simulink library "LIB_CycleControl"  (R2018b)
settings: Solver=VariableStepAuto  StartTime=0.0  StopTime=10.0  RelTol=1e-3
undefined symbols (not defined in the file or in its folder): eActuators, eRespiratorStates, NActuatorActive, nBlowerCmdInit, nBlowerCmdMax, nBlowerCmdMin, nBlowerDecHigh, nBlowerDecMedium, nBlowerIncHigh, nBlowerIncLow, nBlowerIncMedium, NBlowerSpeedIncCorrectionGain, NBlowerValveDerivativeGain, NBlowerValveIntegralGain, NBlowerValveIntegralHighGain, NBlowerValvePropGain, NCyclePerMinMax, NCyclePerMinMin, NMaxPressureSample, NPatientValveDerivativeGain, NPatientValveIntegralGain, NPatientValveIntegralHighGain, NPatientValvePropGain, pBlowerValveOutletOffset, pDiffMaxThdForPlateauPlausibility, pDiffThdForBlowerValveControlActivation, pDiffThdForPatientValveControlActivation, pErrorPlausibilityThd, pErrorThdForHighBlowerDec, pStaticErrorThdForHighBlowerInc, rPIDIntegralMaxTermForBlowerValve, rPIDIntegralMaxTermForPatientValve, rPIDIntegralMinTermForBlowerValve, rPIDIntegralMinTermForPatientValve, tBlowerValveOpen, tDelayBeforeRespiratorCycleStart, tDelayForRespiratorStop, tPatientValveOpen, tPhase1Ofs, tStopInhalationPhase1Min
libraries: simulink x62, simulink_need_slupdate x4, simulink_extras x3
(part 1 of 4)
settings Model: Creator=BRAUL  LastModifiedBy=VITIE

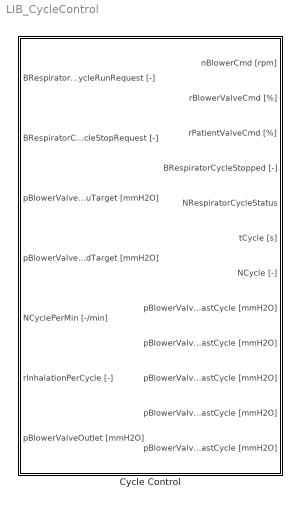
== system LIB_CycleControl ==
  Cycle Control : Subsystem
      settings: AttributesFormatString=%<ReferenceBlock>

== system LIB_CycleControl/Cycle Control ==
  BRespiratorCycleRunRequest [-] : Inport
  BRespiratorCycleStopRequest [-] : Inport  Port=2
  pBlowerValveOutletPlateauTarget [mmH2O] : Inport  Port=3  OutDataTypeStr=single
  pBlowerValveOutletEndTarget [mmH2O] : Inport  Port=4  OutDataTypeStr=single
  NCyclePerMin [-/min] : Inport  Port=5  OutDataTypeStr=single
  rInhalationPerCycle [-] : Inport  Port=6  OutDataTypeStr=single
  pBlowerValveOutlet [mmH2O] : Inport  Port=7  OutDataTypeStr=single
  Compare To Constant : simulink/Logic and Bit Operations/Compare To Constant  relop===  const=eActuators.None  OutDataTypeStr=boolean
  Constant9 : Constant  Value=NActuatorActive  VectorParams1D=off  OutDataTypeStr=Enum: eActuators
  Cycle Control Wrapper : Subsystem
  nBlowerCmd [rpm] : Outport  OutDataTypeStr=single
  rBlowerValveCmd [%] : Outport  Port=2  OutDataTypeStr=single
  rPatientValveCmd [%] : Outport  Port=3  OutDataTypeStr=single
  BRespiratorCycleStopped [-] : Outport  Port=4  OutDataTypeStr=boolean  InitialOutput=0
  NRespiratorCycleStatus : Outport  Port=5
  tCycle [s] : Outport  Port=6
  NCycle [-] : Outport  Port=7
  pBlowerValveOutletPeakLastCycle [mmH2O] : Outport  Port=8
  pBlowerValveOutletPlateauLastCycle [mmH2O] : Outport  Port=9  InitialOutput=0
  pBlowerValveOutletEndLastCycle [mmH2O] : Outport  Port=10
  pBlowerValveOutletPlateauTargetAppliedLastCycle [mmH2O] : Outport  Port=11
  pBlowerValveOutletEndTargetAppliedLastCycle [mmH2O] : Outport  Port=12
  wires:
  Cycle Control Wrapper/7(NCycle [-]) -> NCycle [-]/1
  Cycle Control Wrapper/9(pBlowerValveOutletPlateauLastCycle [mmH2O]) -> pBlowerValveOutletPlateauLastCycle [mmH2O]/1
  Cycle Control Wrapper/8(pBlowerValveOutletPeakLastCycle [mmH2O]) -> pBlowerValveOutletPeakLastCycle [mmH2O]/1
  Cycle Control Wrapper/11(pBlowerValveOutletPlateauTargetAppliedLastCycle [mmH2O]) -> pBlowerValveOutletPlateauTargetAppliedLastCycle [mmH2O]/1
  Cycle Control Wrapper/12(pBlowerValveOutletEndTargetAppliedLastCycle [mmH2O]) -> pBlowerValveOutletEndTargetAppliedLastCycle [mmH2O]/1
  Cycle Control Wrapper/10(pBlowerValveOutletEndLastCycle [mmH2O]) -> pBlowerValveOutletEndLastCycle [mmH2O]/1
  Cycle Control Wrapper/5(NRespiratorCycleStatus) -> NRespiratorCycleStatus/1
  Cycle Control Wrapper/6(tCycle [s]) -> tCycle [s]/1
  BRespiratorCycleStopRequest [-]/1 -> Cycle Control Wrapper/2(BRespiratorCycleStopRequest [-])
  BRespiratorCycleRunRequest [-]/1 -> Cycle Control Wrapper/1(BRespiratorCycleRunRequest [-])
  Cycle Control Wrapper/4(BRespiratorCycleStopped [-]) -> BRespiratorCycleStopped [-]/1
  Cycle Control Wrapper/1(nBlowerCmd [rpm]) -> nBlowerCmd [rpm]/1
  Cycle Control Wrapper/2(rBlowerValveCmd [%]) -> rBlowerValveCmd [%]/1
  Cycle Control Wrapper/3(rPatientValveCmd [%]) -> rPatientValveCmd [%]/1
  pBlowerValveOutletPlateauTarget [mmH2O]/1 -> Cycle Control Wrapper/3(pBlowerValveOutletPlateauTarget [mmH2O])
  pBlowerValveOutletEndTarget [mmH2O]/1 -> Cycle Control Wrapper/4(pBlowerValveOutletEndTarget [mmH2O])
  NCyclePerMin [-/min]/1 -> Cycle Control Wrapper/5(NCyclePerMin [-/min])
  rInhalationPerCycle [-]/1 -> Cycle Control Wrapper/6(rInhalationPerCycle [-])
  pBlowerValveOutlet [mmH2O]/1 -> Cycle Control Wrapper/7(pBlowerValveOutlet [mmH2O])
  Compare To Constant/1 -> Cycle Control Wrapper/Enable
  Constant9/1 -> Compare To Constant/1

== system LIB_CycleControl/Cycle Control/Cycle Control Wrapper ==
  BRespiratorCycleRunRequest [-] : Inport
  BRespiratorCycleStopRequest [-] : Inport  Port=2
  pBlowerValveOutletPlateauTarget [mmH2O] : Inport  Port=3  OutDataTypeStr=single
  pBlowerValveOutletEndTarget [mmH2O] : Inport  Port=4  OutDataTypeStr=single
  NCyclePerMin [-/min] : Inport  Port=5  OutDataTypeStr=single
  rInhalationPerCycle [-] : Inport  Port=6  OutDataTypeStr=single
  pBlowerValveOutlet [mmH2O] : Inport  Port=7  OutDataTypeStr=single
  Enable : EnablePort  StatesWhenEnabling=reset
  Cycle pController : Subsystem
  nBlowerCmd [rpm] : Outport  OutDataTypeStr=single  InitialOutput=0
  rBlowerValveCmd [%] : Outport  Port=2  OutDataTypeStr=single  InitialOutput=0
  rPatientValveCmd [%] : Outport  Port=3  OutDataTypeStr=single  InitialOutput=0
  BRespiratorCycleStopped [-] : Outport  Port=4  InitialOutput=0
  NRespiratorCycleStatus : Outport  Port=5
  tCycle [s] : Outport  Port=6
  NCycle [-] : Outport  Port=7
  pBlowerValveOutletPeakLastCycle [mmH2O] : Outport  Port=8
  pBlowerValveOutletPlateauLastCycle [mmH2O] : Outport  Port=9  InitialOutput=0
  pBlowerValveOutletEndLastCycle [mmH2O] : Outport  Port=10
  pBlowerValveOutletPlateauTargetAppliedLastCycle [mmH2O] : Outport  Port=11
  pBlowerValveOutletEndTargetAppliedLastCycle [mmH2O] : Outport  Port=12
  wires:
  Cycle pController/7(NCycle [-]) -> NCycle [-]/1
  Cycle pController/11(pBlowerValveOutletEndTargetAppliedLastCycle [mmH2O]) -> pBlowerValveOutletEndTargetAppliedLastCycle [mmH2O]/1
  Cycle pController/12(pBlowerValveOutletPlateauTargetAppliedLastCycle [mmH2O]) -> pBlowerValveOutletPlateauTargetAppliedLastCycle [mmH2O]/1
  Cycle pController/10(pBlowerValveOutletPlateauLastCycle [mmH2O]) -> pBlowerValveOutletPlateauLastCycle [mmH2O]/1
  Cycle pController/9(pBlowerValveOutletEndLastCycle [mmH2O]) -> pBlowerValveOutletEndLastCycle [mmH2O]/1
  Cycle pController/8(pBlowerValveOutletPeakLastCycle [mmH2O]) -> pBlowerValveOutletPeakLastCycle [mmH2O]/1
  Cycle pController/6(tCycle [s]) -> tCycle [s]/1
  Cycle pController/5(NRespiratorCycleStatus) -> NRespiratorCycleStatus/1
  BRespiratorCycleRunRequest [-]/1 -> Cycle pController/1(BRespiratorCycleRunRequest [-])
  BRespiratorCycleStopRequest [-]/1 -> Cycle pController/2(BRespiratorCycleStopRequest [-])
  Cycle pController/4(BRespiratorCycleStopped [-]) -> BRespiratorCycleStopped [-]/1
  pBlowerValveOutletEndTarget [mmH2O]/1 -> Cycle pController/4(pBlowerValveOutletEndTarget [mmH2O])
  Cycle pController/2(rBlowerValveCmd [%]) -> rBlowerValveCmd [%]/1
  Cycle pController/1(nBlowerCmd [rpm]) -> nBlowerCmd [rpm]/1
  NCyclePerMin [-/min]/1 -> Cycle pController/5(NCyclePerMin [-/min])
  pBlowerValveOutletPlateauTarget [mmH2O]/1 -> Cycle pController/3(pBlowerValveOutletPlateauTarget [mmH2O])
  rInhalationPerCycle [-]/1 -> Cycle pController/6(rInhalationPerCycle [-])
  Cycle pController/3(rPatientValveCmd [%]) -> rPatientValveCmd [%]/1
  pBlowerValveOutlet [mmH2O]/1 -> Cycle pController/7(pBlowerValveOutlet [mmH2O])

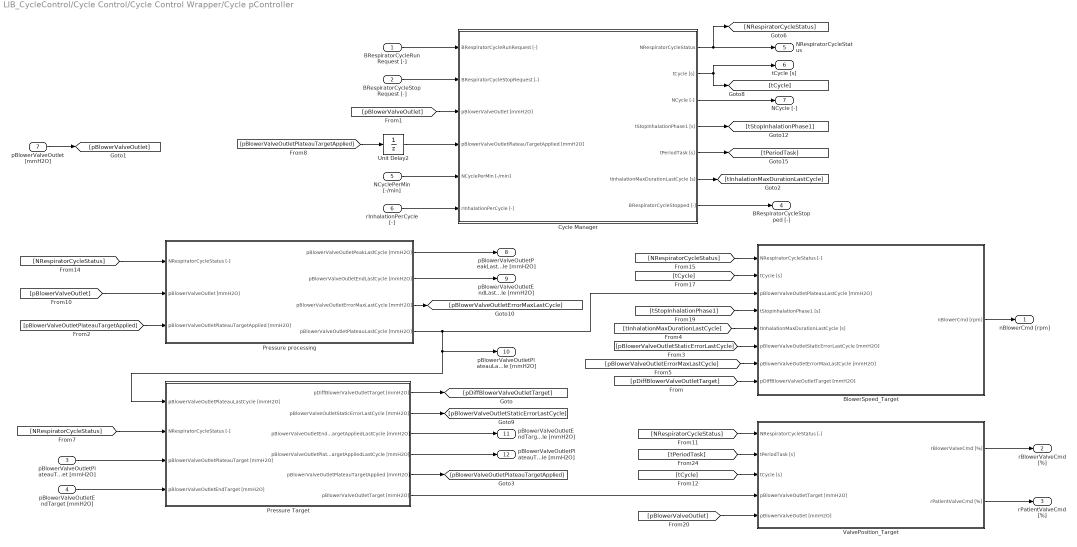
== system LIB_CycleControl/Cycle Control/Cycle Control Wrapper/Cycle pController ==
  BRespiratorCycleRunRequest [-] : Inport
  BRespiratorCycleStopRequest [-] : Inport  Port=2
  pBlowerValveOutletPlateauTarget [mmH2O] : Inport  Port=3
  pBlowerValveOutletEndTarget [mmH2O] : Inport  Port=4
  NCyclePerMin [-/min] : Inport  Port=5
  rInhalationPerCycle [-] : Inport  Port=6
  pBlowerValveOutlet [mmH2O] : Inport  Port=7
  BlowerSpeed_Target : Subsystem
  Cycle Manager : Subsystem
  Pressure Target : Subsystem
  Pressure processing : Subsystem
  Unit Delay2 : UnitDelay  SampleTime=-1
      settings: AttributesFormatString=%<InitialCondition>
  ValvePosition_Target : Subsystem
  nBlowerCmd [rpm] : Outport  InitialOutput=0
  rBlowerValveCmd [%] : Outport  Port=2  InitialOutput=0
  rPatientValveCmd [%] : Outport  Port=3  InitialOutput=0
  BRespiratorCycleStopped [-] : Outport  Port=4  InitialOutput=0
  NRespiratorCycleStatus : Outport  Port=5
  tCycle [s] : Outport  Port=6
  NCycle [-] : Outport  Port=7
  pBlowerValveOutletPeakLastCycle [mmH2O] : Outport  Port=8
  pBlowerValveOutletEndLastCycle [mmH2O] : Outport  Port=9
  pBlowerValveOutletPlateauLastCycle [mmH2O] : Outport  Port=10  InitialOutput=0
  pBlowerValveOutletEndTargetAppliedLastCycle [mmH2O] : Outport  Port=11
  pBlowerValveOutletPlateauTargetAppliedLastCycle [mmH2O] : Outport  Port=12
  wires:
  Cycle Manager/3(NCycle [-]) -> NCycle [-]/1
  Pressure processing/2(pBlowerValveOutletEndLastCycle [mmH2O]) -> pBlowerValveOutletEndLastCycle [mmH2O]/1
  Pressure processing/1(pBlowerValveOutletPeakLastCycle [mmH2O]) -> pBlowerValveOutletPeakLastCycle [mmH2O]/1
  Pressure processing/4(pBlowerValveOutletPlateauLastCycle [mmH2O]) -> BlowerSpeed_Target/3(pBlowerValveOutletPlateauLastCycle [mmH2O]), pBlowerValveOutletPlateauLastCycle [mmH2O]/1, Pressure Target/1(pBlowerValveOutletPlateauLastCycle [mmH2O])
  Pressure processing/3(pBlowerValveOutletErrorMaxLastCycle [mmH2O]) -> [pBlowerValveOutletErrorMaxLastCycle]
  Pressure Target/4(pBlowerValveOutletPlateauTargetAppliedLastCycle [mmH2O]) -> pBlowerValveOutletPlateauTargetAppliedLastCycle [mmH2O]/1
  Pressure Target/3(pBlowerValveOutletEndTargetAppliedLastCycle [mmH2O]) -> pBlowerValveOutletEndTargetAppliedLastCycle [mmH2O]/1
  Pressure Target/5(pBlowerValveOutletPlateauTargetApplied [mmH2O]) -> [pBlowerValveOutletPlateauTargetApplied]
  Pressure Target/1(pDiffBlowerValveOutletTarget [mmH2O]) -> [pDiffBlowerValveOutletTarget]
  [pBlowerValveOutletErrorMaxLastCycle] -> BlowerSpeed_Target/7(pBlowerValveOutletErrorMaxLastCycle [mmH2O])
  [pDiffBlowerValveOutletTarget] -> BlowerSpeed_Target/8(pDiffBlowerValveOutletTarget [mmH2O])
  [pBlowerValveOutletPlateauTargetApplied] -> Pressure processing/3(pBlowerValveOutletPlateauTargetApplied [mmH2O])
  [tCycle] -> ValvePosition_Target/3(tCycle [s])
  BRespiratorCycleRunRequest [-]/1 -> Cycle Manager/1(BRespiratorCycleRunRequest [-])
  BRespiratorCycleStopRequest [-]/1 -> Cycle Manager/2(BRespiratorCycleStopRequest [-])
  Cycle Manager/7(BRespiratorCycleStopped [-]) -> BRespiratorCycleStopped [-]/1
  Cycle Manager/6(tInhalationMaxDurationLastCycle [s]) -> [tInhalationMaxDurationLastCycle]
  Cycle Manager/5(tPeriodTask [s]) -> [tPeriodTask]
  Pressure Target/6(pBlowerValveOutletTarget [mmH2O]) -> ValvePosition_Target/4(pBlowerValveOutletTarget [mmH2O])
  Unit Delay2/1 -> Cycle Manager/4(pBlowerValveOutletPlateauTargetApplied [mmH2O])
  [pBlowerValveOutlet] -> Cycle Manager/3(pBlowerValveOutlet [mmH2O])
  Cycle Manager/4(tStopInhalationPhase1 [s]) -> [tStopInhalationPhase1]
  Cycle Manager/2(tCycle [s]) -> tCycle [s]/1, [tCycle]
  Cycle Manager/1(NRespiratorCycleStatus) -> NRespiratorCycleStatus/1, [NRespiratorCycleStatus]
  rInhalationPerCycle [-]/1 -> Cycle Manager/6(rInhalationPerCycle [-])
  NCyclePerMin [-/min]/1 -> Cycle Manager/5(NCyclePerMin [-/min])
  [pBlowerValveOutletPlateauTargetApplied] -> Unit Delay2/1
  pBlowerValveOutlet [mmH2O]/1 -> [pBlowerValveOutlet]
  [tPeriodTask] -> ValvePosition_Target/2(tPeriodTask [s])
  [pBlowerValveOutletStaticErrorLastCycle] -> BlowerSpeed_Target/6("pBlowerValveOutletStaticErrorLastCycle [mmH2O] ")
  [tInhalationMaxDurationLastCycle] -> BlowerSpeed_Target/5(tInhalationMaxDurationLastCycle [s])
  [tStopInhalationPhase1] -> BlowerSpeed_Target/4(tStopInhalationPhase1 [s])
  Pressure Target/2(pBlowerValveOutletStaticErrorLastCycle [mmH2O]) -> [pBlowerValveOutletStaticErrorLastCycle]
  pBlowerValveOutletPlateauTarget [mmH2O]/1 -> Pressure Target/3(pBlowerValveOutletPlateauTarget [mmH2O])
  [NRespiratorCycleStatus] -> Pressure Target/2(NRespiratorCycleStatus [-])
  pBlowerValveOutletEndTarget [mmH2O]/1 -> Pressure Target/4(pBlowerValveOutletEndTarget [mmH2O])
  [NRespiratorCycleStatus] -> Pressure processing/1(NRespiratorCycleStatus [-])
  [pBlowerValveOutlet] -> Pressure processing/2(pBlowerValveOutlet [mmH2O])
  [pBlowerValveOutlet] -> ValvePosition_Target/5(pBlowerValveOutlet [mmH2O])
  [NRespiratorCycleStatus] -> ValvePosition_Target/1(NRespiratorCycleStatus [-])
  [tCycle] -> BlowerSpeed_Target/2(tCycle [s])
  [NRespiratorCycleStatus] -> BlowerSpeed_Target/1(NRespiratorCycleStatus [-])
  ValvePosition_Target/2(rPatientValveCmd [%]) -> rPatientValveCmd [%]/1
  ValvePosition_Target/1(rBlowerValveCmd [%]) -> rBlowerValveCmd [%]/1
  BlowerSpeed_Target/1(nBlowerCmd [rpm]) -> nBlowerCmd [rpm]/1

== system LIB_CycleControl/Cycle Control/Cycle Control Wrapper/Cycle pController/BlowerSpeed_Target ==
  NRespiratorCycleStatus [-] : Inport
  tCycle [s] : Inport  Port=2
  pBlowerValveOutletPlateauLastCycle [mmH2O] : Inport  Port=3
  tStopInhalationPhase1 [s] : Inport  Port=4
  tInhalationMaxDurationLastCycle [s] : Inport  Port=5
  "pBlowerValveOutletStaticErrorLastCycle [mmH2O] " : Inport  Port=6
  pBlowerValveOutletErrorMaxLastCycle [mmH2O] : Inport  Port=7
  pDiffBlowerValveOutletTarget [mmH2O] : Inport  Port=8
  Compare To Constant1 : simulink/Logic and Bit Operations/Compare To Constant  relop===  const=eRespiratorStates.NRespiratorStart  OutDataTypeStr=boolean
  Compare To Constant2 : simulink/Logic and Bit Operations/Compare To Constant  relop===  const=eRespiratorStates.NRespiratorInInhalationPhase1  OutDataTypeStr=boolean
  Compare To Constant3 : simulink/Logic and Bit Operations/Compare To Constant  relop===  const=eRespiratorStates.NRespiratorStop  OutDataTypeStr=boolean
  CycleStartComputation : Subsystem
  Data Type Conversion : DataTypeConversion
  Detect Increase : simulink/Logic and Bit Operations/Detect Increase  vinit=0.0  OutDataTypeStr=boolean
  If : If  NumInputs=3  IfExpression=u1 ~= 0  ElseIfExpressions=u2 ~= 0,u3 ~= 0  ShowElse=off
  Merge : Merge  Inputs=3  InitialOutput=0
  START : Subsystem
  STOP : Subsystem
  Unit Delay1 : UnitDelay  SampleTime=-1
      settings: AttributesFormatString=%<InitialCondition>
  Unit Delay2 : UnitDelay  SampleTime=-1
      settings: AttributesFormatString=%<InitialCondition>
  nBlowerCmd [rpm] : Outport
  wires:
  Data Type Conversion/1 -> nBlowerCmd [rpm]/1
  pDiffBlowerValveOutletTarget [mmH2O]/1 -> CycleStartComputation/6(pDiffBlowerValveOutletTarget [mmH2O])
  pBlowerValveOutletErrorMaxLastCycle [mmH2O]/1 -> CycleStartComputation/5(pBlowerValveOutletErrorMaxLastCycle [mmH2O])
  CycleStartComputation/1(nBlowerCmd [rpm]) -> Merge/3
  STOP/1(nBlowerCmd [rpm]) -> Merge/2
  [tCycle] -> START/1(tCycle [s])
  If/3 -> CycleStartComputation/Action
  If/2 -> STOP/Action
  Compare To Constant3/1 -> If/2
  Unit Delay2/1 -> CycleStartComputation/2(tStopInhalationPhase1LastCycle [s])
  Merge/1 -> Unit Delay1/1, Data Type Conversion/1
  START/1(nBlowerCmd [rpm]) -> Merge/1
  Detect Increase/1 -> If/3
  If/1 -> START/Action
  Compare To Constant1/1 -> If/1
  Unit Delay1/1 -> CycleStartComputation/7(nBlowerCmdPrev [rpm])
  "pBlowerValveOutletStaticErrorLastCycle [mmH2O] "/1 -> CycleStartComputation/4("pBlowerValveOutletStaticErrorLastCycle [mmH2O] ")
  tInhalationMaxDurationLastCycle [s]/1 -> CycleStartComputation/3(tInhalationMaxDurationLastCycle [s])
  tStopInhalationPhase1 [s]/1 -> Unit Delay2/1
  pBlowerValveOutletPlateauLastCycle [mmH2O]/1 -> CycleStartComputation/1(pBlowerValveOutletPlateauLastCycle [mmH2O])
  NRespiratorCycleStatus [-]/1 -> [NRespiratorCycleStatus]
  [NRespiratorCycleStatus] -> Compare To Constant3/1, Compare To Constant2/1, Compare To Constant1/1
  Compare To Constant2/1 -> Detect Increase/1
  tCycle [s]/1 -> [tCycle]

== system LIB_CycleControl/Cycle Control/Cycle Control Wrapper/Cycle pController/Cycle Manager ==
  BRespiratorCycleRunRequest [-] : Inport
  BRespiratorCycleStopRequest [-] : Inport  Port=2
  pBlowerValveOutlet [mmH2O] : Inport  Port=3
  pBlowerValveOutletPlateauTargetApplied [mmH2O] : Inport  Port=4
  NCyclePerMin [-/min] : Inport  Port=5
  rInhalationPerCycle [-] : Inport  Port=6
  1 : Constant  OutDataTypeStr=single
  Constant3 : Constant  Value=tDelayForRespiratorStop  OutDataTypeStr=single
  Constant4 : Constant  Value=tDelayBeforeRespiratorCycleStart  OutDataTypeStr=single
  Constant9 : Constant  Value=pBlowerValveOutletOffset  OutDataTypeStr=single
  Data Store Write1 : DataStoreWrite  DataStoreName=tCycle
  Data Store Write2 : DataStoreWrite  DataStoreName=NCycle
  Data Store Write3 : DataStoreWrite  DataStoreName=NRespiratorCycleStatus
  Data Store Write4 : DataStoreWrite  DataStoreName=tStopInhalationPhase1
  Data Store Write5 : DataStoreWrite  DataStoreName=BRespiratorCycleStopped
  Respiratory Cycle Management : Stateflow chart  TreatAsAtomicUnit=on
  Timing Setup : Subsystem
  Weighted Sample Time : SampleTimeMath  TsampMathOp=Ts Only  OutDataTypeStr=Inherit: Inherit via back propagation
  NRespiratorCycleStatus : Outport
  tCycle [s] : Outport  Port=2
  NCycle [-] : Outport  Port=3
  tStopInhalationPhase1 [s] : Outport  Port=4
  tPeriodTask [s] : Outport  Port=5
  tInhalationMaxDurationLastCycle [s] : Outport  Port=6
  BRespiratorCycleStopped [-] : Outport  Port=7
  wires:
  Constant3/1 -> Respiratory Cycle Management/10(tDelayForRespiratorStop)
  Constant4/1 -> Respiratory Cycle Management/9(tDelayBeforeRespiratorCycleStart)
  Constant9/1 -> Respiratory Cycle Management/8(pBlowerValveOutletOffset)
  BRespiratorCycleStopRequest [-]/1 -> Respiratory Cycle Management/2(BRespiratorCycleStopRequest)
  BRespiratorCycleRunRequest [-]/1 -> Respiratory Cycle Management/1(BRespiratorCycleRunRequest)
  Respiratory Cycle Management/5(BRespiratorCycleStopped) -> BRespiratorCycleStopped [-]/1, Data Store Write5/1  "BRespiratorCycleStopped"
  Timing Setup/3(tInhalationMaxDurationLastCycle [s]) -> tInhalationMaxDurationLastCycle [s]/1
  Respiratory Cycle Management/1(NRespiratorCycleStatus) -> NRespiratorCycleStatus/1, Data Store Write3/1  "NRespiratorCycleStatus"
  Respiratory Cycle Management/3(NCycle) -> Data Store Write2/1, NCycle [-]/1  "NCycle"
  Timing Setup/2(tInhalationMaxDuration [s]) -> [tInhalationMaxDuration]
  [tInhalationMaxDuration] -> Respiratory Cycle Management/3(tInhalationMaxDuration)
  Respiratory Cycle Management/4(tStopInhalationPhase1) -> tStopInhalationPhase1 [s]/1, Data Store Write4/1  "tStopInhalationPhase1"
  NCyclePerMin [-/min]/1 -> Timing Setup/1(NCyclePerMin [-/min])
  Respiratory Cycle Management/6(fCallCycleComputation()) -> Timing Setup/Trigger
  [tCycleMaxDuration] -> Respiratory Cycle Management/4(tCycleMaxDuration)
  1/1 -> Weighted Sample Time/1
  pBlowerValveOutlet [mmH2O]/1 -> [pBlowerValveOutlet]
  [pBlowerValveOutlet] -> Respiratory Cycle Management/6(pBlowerValveOutlet)
  Timing Setup/1(tCycleMaxDuration [s]) -> [tCycleMaxDuration]
  pBlowerValveOutletPlateauTargetApplied [mmH2O]/1 -> Respiratory Cycle Management/7(pBlowerValveOutletPlateauTargetApplied)
  rInhalationPerCycle [-]/1 -> Timing Setup/2(rInhalationPerCycle [-])
  Respiratory Cycle Management/2(tCycle) -> tCycle [s]/1, Data Store Write1/1  "tCycle"
  Weighted Sample Time/1 -> tPeriodTask [s]/1, Respiratory Cycle Management/5(tSample)

== system LIB_CycleControl/Cycle Control/Cycle Control Wrapper/Cycle pController/Pressure Target ==
  pBlowerValveOutletPlateauLastCycle [mmH2O] : Inport
  NRespiratorCycleStatus [-] : Inport  Port=2
  pBlowerValveOutletPlateauTarget [mmH2O] : Inport  Port=3
  pBlowerValveOutletEndTarget [mmH2O] : Inport  Port=4
  CycleStartComputation : Subsystem
  Data Store Write4 : DataStoreWrite  DataStoreName=pBlowerValveOutletTarget
  InCycleComputation : Subsystem
  pDiffBlowerValveOutletTarget [mmH2O] : Outport
  pBlowerValveOutletStaticErrorLastCycle [mmH2O] : Outport  Port=2
  pBlowerValveOutletEndTargetAppliedLastCycle [mmH2O] : Outport  Port=3
  pBlowerValveOutletPlateauTargetAppliedLastCycle [mmH2O] : Outport  Port=4
  pBlowerValveOutletPlateauTargetApplied [mmH2O] : Outport  Port=5
  pBlowerValveOutletTarget [mmH2O] : Outport  Port=6
  wires:
  CycleStartComputation/1(pDiffBlowerValveOutletTarget [mmH2O]) -> pDiffBlowerValveOutletTarget [mmH2O]/1
  CycleStartComputation/2(pBlowerValveOutletStaticErrorLastCycle [mmH2O]) -> pBlowerValveOutletStaticErrorLastCycle [mmH2O]/1
  CycleStartComputation/4(pBlowerValveOutletPlateauTargetAppliedLastCycle [mmH2O]) -> pBlowerValveOutletPlateauTargetAppliedLastCycle [mmH2O]/1
  CycleStartComputation/3(pBlowerValveOutletEndTargetAppliedLastCycle [mmH2O]) -> pBlowerValveOutletEndTargetAppliedLastCycle [mmH2O]/1
  CycleStartComputation/5(pBlowerValveOutletEndTargetApplied [mmH2O]) -> InCycleComputation/2(pBlowerValveOutletEndTargetApplied [mmH2O])
  [NRespiratorCycleStatus] -> CycleStartComputation/1(NRespiratorCycleStatus [-])
  pBlowerValveOutletEndTarget [mmH2O]/1 -> CycleStartComputation/4(pBlowerValveOutletEndTarget [mmH2O])
  pBlowerValveOutletPlateauTarget [mmH2O]/1 -> CycleStartComputation/2(pBlowerValveOutletPlateauTarget [mmH2O])
  pBlowerValveOutletPlateauLastCycle [mmH2O]/1 -> CycleStartComputation/3(pBlowerValveOutletPlateauLastCycle [mmH2O])
  [NRespiratorCycleStatus] -> InCycleComputation/1(NRespiratorCycleStatus [-])
  CycleStartComputation/6(pBlowerValveOutletPlateauTargetApplied [mmH2O]) -> InCycleComputation/3(pBlowerValveOutletPlateauTargetApplied [mmH2O]), pBlowerValveOutletPlateauTargetApplied [mmH2O]/1
  NRespiratorCycleStatus [-]/1 -> [NRespiratorCycleStatus]
  InCycleComputation/1(pBlowerValveOutletTarget [mmH2O]) -> pBlowerValveOutletTarget [mmH2O]/1, Data Store Write4/1  "pBlowerValveOutletTarget"

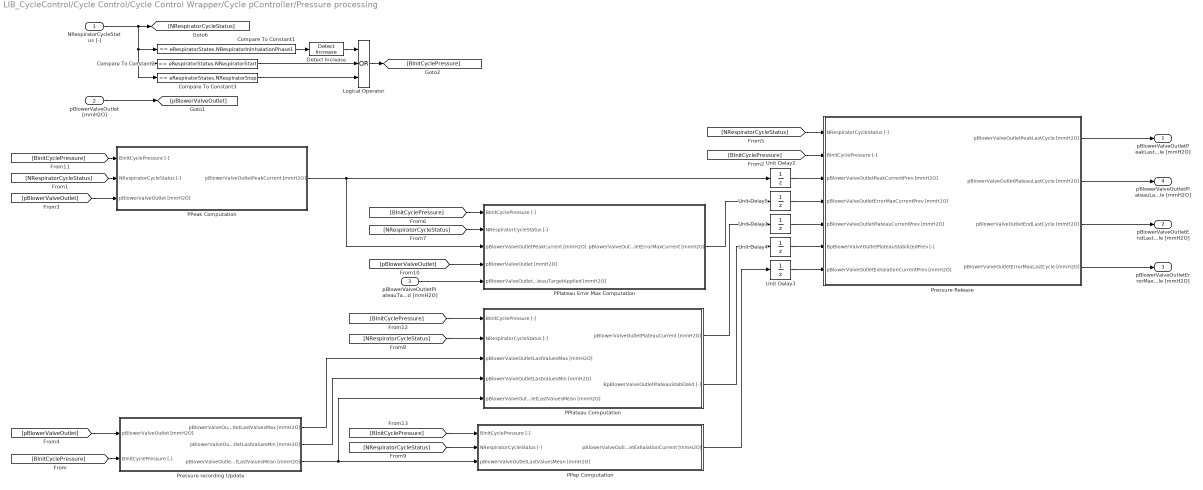
== system LIB_CycleControl/Cycle Control/Cycle Control Wrapper/Cycle pController/Pressure processing ==
  NRespiratorCycleStatus [-] : Inport
  pBlowerValveOutlet [mmH2O] : Inport  Port=2
  pBlowerValveOutletPlateauTargetApplied [mmH2O] : Inport  Port=3
  Compare To Constant1 : simulink/Logic and Bit Operations/Compare To Constant  relop===  const=eRespiratorStates.NRespiratorInInhalationPhase1  OutDataTypeStr=boolean
  Compare To Constant2 : simulink/Logic and Bit Operations/Compare To Constant  relop===  const=eRespiratorStates.NRespiratorStart  OutDataTypeStr=boolean
  Compare To Constant3 : simulink/Logic and Bit Operations/Compare To Constant  relop===  const=eRespiratorStates.NRespiratorStop  OutDataTypeStr=boolean
  Detect Increase : simulink/Logic and Bit Operations/Detect Increase  vinit=0.0  OutDataTypeStr=boolean
  Logical Operator : Logic  Operator=OR  Inputs=3  AllPortsSameDT=off  OutDataTypeStr=boolean
  PPeak Computation : Subsystem
  PPep Computation : Subsystem
  PPlateau Computation : Subsystem
  PPlateau Error Max Computation : Subsystem
  "Pressure Release " : Subsystem
  Pressure recording Update : Subsystem
  Unit Delay{1..3,5} (4 alike) : UnitDelay  SampleTime=-1
      settings: AttributesFormatString=%<InitialCondition>
  Unit Delay4 : UnitDelay  InitialCondition=1  SampleTime=-1
      settings: AttributesFormatString=%<InitialCondition>
  pBlowerValveOutletPeakLastCycle [mmH2O] : Outport
  pBlowerValveOutletEndLastCycle [mmH2O] : Outport  Port=2
  pBlowerValveOutletErrorMaxLastCycle [mmH2O] : Outport  Port=3  InitialOutput=0
  pBlowerValveOutletPlateauLastCycle [mmH2O] : Outport  Port=4  InitialOutput=0
  wires:
  "Pressure Release "/1(pBlowerValveOutletPeakLastCycle [mmH2O]) -> pBlowerValveOutletPeakLastCycle [mmH2O]/1
  "Pressure Release "/2(pBlowerValveOutletPlateauLastCycle [mmH2O]) -> pBlowerValveOutletPlateauLastCycle [mmH2O]/1
  "Pressure Release "/3(pBlowerValveOutletEndLastCycle [mmH2O]) -> pBlowerValveOutletEndLastCycle [mmH2O]/1
  "Pressure Release "/4(pBlowerValveOutletErrorMaxLastCycle [mmH2O]) -> pBlowerValveOutletErrorMaxLastCycle [mmH2O]/1
  PPlateau Error Max Computation/1(pBlowerValveOutletErrorMaxCurrent [mmH2O]) -> Unit Delay5/1
  Unit Delay5/1 -> "Pressure Release "/4(pBlowerValveOutletErrorMaxCurrentPrev [mmH2O])
  PPlateau Computation/2(BpBlowerValveOutletPlateauStabilized [-]) -> Unit Delay4/1
  Unit Delay4/1 -> "Pressure Release "/6(BpBlowerValveOutletPlateauStabilizedPrev [-])
  pBlowerValveOutletPlateauTargetApplied [mmH2O]/1 -> PPlateau Error Max Computation/5(pBlowerValveOutletPlateauTargetApplied [mmH2O])
  [pBlowerValveOutlet] -> PPlateau Error Max Computation/4(pBlowerValveOutlet [mmH2O])
  [NRespiratorCycleStatus] -> PPlateau Error Max Computation/2(NRespiratorCycleStatus [-])
  [BInitCyclePressure] -> PPlateau Error Max Computation/1(BInitCyclePressure [-])
  Pressure recording Update/2(pBlowerValveOutletLastValuesMin [mmH2O]) -> PPlateau Computation/4(pBlowerValveOutletLastValuesMin [mmH2O])
  Pressure recording Update/1(pBlowerValveOutletLastValuesMax [mmH2O]) -> PPlateau Computation/3(pBlowerValveOutletLastValuesMax [mmH2O])
  [BInitCyclePressure] -> "Pressure Release "/2(BInitCyclePressure [-])
  Unit Delay3/1 -> "Pressure Release "/7(pBlowerValveOutletExhalationCurrentPrev [mmH2O])
  PPep Computation/1(pBlowerValveOutletExhalationCurrent [mmH2O]) -> Unit Delay3/1
  Unit Delay1/1 -> "Pressure Release "/5(pBlowerValveOutletPlateauCurrentPrev [mmH2O])
  Unit Delay2/1 -> "Pressure Release "/3(pBlowerValveOutletPeakCurrentPrev [mmH2O])
  PPlateau Computation/1(pBlowerValveOutletPlateauCurrent [mmH2O]) -> Unit Delay1/1
  PPeak Computation/1(pBlowerValveOutletPeakCurrent [mmH2O]) -> Unit Delay2/1, PPlateau Error Max Computation/3(pBlowerValveOutletPeakCurrent [mmH2O])
  [BInitCyclePressure] -> Pressure recording Update/2(BInitCyclePressure [-])
  [BInitCyclePressure] -> PPep Computation/1(BInitCyclePressure [-])
  [BInitCyclePressure] -> PPlateau Computation/1(BInitCyclePressure [-])
  [BInitCyclePressure] -> PPeak Computation/1(BInitCyclePressure [-])
  NRespiratorCycleStatus [-]/1 -> [NRespiratorCycleStatus], Compare To Constant3/1, Compare To Constant2/1, Compare To Constant1/1
  Compare To Constant1/1 -> Detect Increase/1
  [NRespiratorCycleStatus] -> PPep Computation/2(NRespiratorCycleStatus [-])
  [NRespiratorCycleStatus] -> PPlateau Computation/2(NRespiratorCycleStatus [-])
  Pressure recording Update/3(pBlowerValveOutletLastValuesMean [mmH2O]) -> PPlateau Computation/5(pBlowerValveOutletLastValuesMean [mmH2O]), PPep Computation/3(pBlowerValveOutletLastValuesMean [mmH2O])
  [pBlowerValveOutlet] -> Pressure recording Update/1(pBlowerValveOutlet [mmH2O])
  [pBlowerValveOutlet] -> PPeak Computation/3(pBlowerValveOutlet [mmH2O])
  [NRespiratorCycleStatus] -> PPeak Computation/2(NRespiratorCycleStatus [-])
  pBlowerValveOutlet [mmH2O]/1 -> [pBlowerValveOutlet]
  Detect Increase/1 -> Logical Operator/1
  Compare To Constant2/1 -> Logical Operator/2
  Compare To Constant3/1 -> Logical Operator/3
  Logical Operator/1 -> [BInitCyclePressure]
  [NRespiratorCycleStatus] -> "Pressure Release "/1(NRespiratorCycleStatus [-])

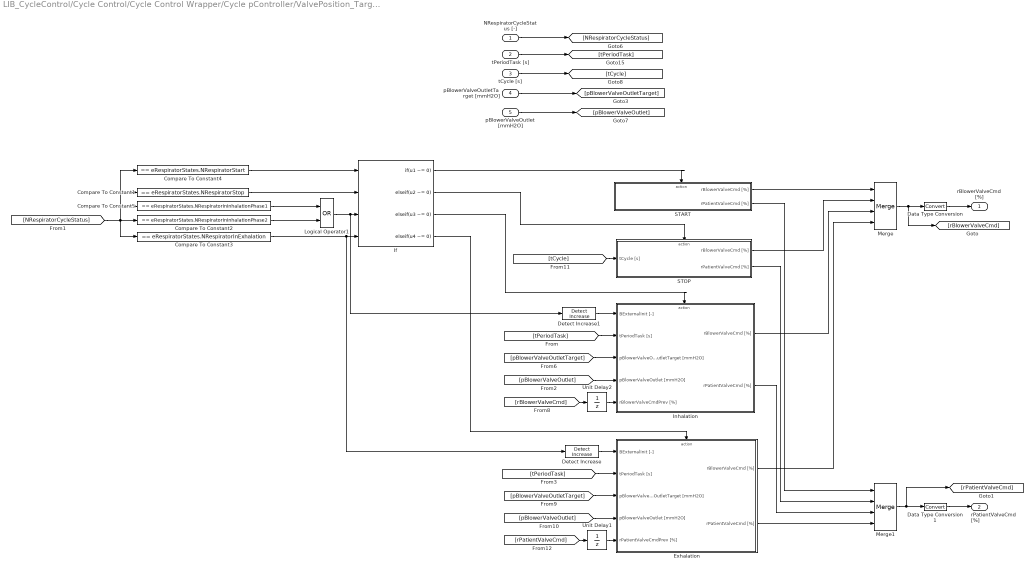
== system LIB_CycleControl/Cycle Control/Cycle Control Wrapper/Cycle pController/ValvePosition_Target ==
  NRespiratorCycleStatus [-] : Inport
  tPeriodTask [s] : Inport  Port=2
  tCycle [s] : Inport  Port=3
  pBlowerValveOutletTarget [mmH2O] : Inport  Port=4
  pBlowerValveOutlet [mmH2O] : Inport  Port=5
  Compare To Constant1 : simulink/Logic and Bit Operations/Compare To Constant  relop===  const=eRespiratorStates.NRespiratorStop  OutDataTypeStr=boolean
  Compare To Constant2 : simulink/Logic and Bit Operations/Compare To Constant  relop===  const=eRespiratorStates.NRespiratorInInhalationPhase2  OutDataTypeStr=boolean
  Compare To Constant3 : simulink/Logic and Bit Operations/Compare To Constant  relop===  const=eRespiratorStates.NRespiratorInExhalation  OutDataTypeStr=boolean
  Compare To Constant4 : simulink/Logic and Bit Operations/Compare To Constant  relop===  const=eRespiratorStates.NRespiratorStart  OutDataTypeStr=boolean
  Compare To Constant5 : simulink/Logic and Bit Operations/Compare To Constant  relop===  const=eRespiratorStates.NRespiratorInInhalationPhase1  OutDataTypeStr=boolean
  Data Type Conversion : DataTypeConversion
  Data Type Conversion1 : DataTypeConversion
  Detect Increase : simulink/Logic and Bit Operations/Detect Increase  vinit=0.0  OutDataTypeStr=boolean
  Detect Increase1 : simulink/Logic and Bit Operations/Detect Increase  vinit=0.0  OutDataTypeStr=boolean
  Exhalation : Subsystem
  If : If  NumInputs=4  IfExpression=u1 ~= 0  ElseIfExpressions=u2 ~= 0,u3 ~= 0,u4 ~= 0  ShowElse=off
  Inhalation : Subsystem
  Logical Operator1 : Logic  Operator=OR  AllPortsSameDT=off  OutDataTypeStr=boolean
  Merge : Merge  Inputs=4  InitialOutput=0
  Merge1 : Merge  Inputs=4  InitialOutput=0
  START : Subsystem
  STOP : Subsystem
  Unit Delay1 : UnitDelay  SampleTime=-1
  Unit Delay2 : UnitDelay  SampleTime=-1
  rBlowerValveCmd [%] : Outport
  rPatientValveCmd [%] : Outport  Port=2
  wires:
  Data Type Conversion1/1 -> rPatientValveCmd [%]/1
  Data Type Conversion/1 -> rBlowerValveCmd [%]/1
  If/3 -> Inhalation/Action
  Exhalation/2(rPatientValveCmd [%]) -> Merge1/4
  Inhalation/2(rPatientValveCmd [%]) -> Merge1/3
  STOP/2(rPatientValveCmd [%]) -> Merge1/2
  START/2(rPatientValveCmd [%]) -> Merge1/1
  Exhalation/1(rBlowerValveCmd [%]) -> Merge/4
  Inhalation/1(rBlowerValveCmd [%]) -> Merge/3
  STOP/1(rBlowerValveCmd [%]) -> Merge/2
  START/1(rBlowerValveCmd [%]) -> Merge/1
  If/4 -> Exhalation/Action
  If/2 -> STOP/Action
  [tCycle] -> STOP/1(tCycle [s])
  tCycle [s]/1 -> [tCycle]
  If/1 -> START/Action
  Compare To Constant3/1 -> If/4, Detect Increase/1
  Logical Operator1/1 -> If/3, Detect Increase1/1
  Compare To Constant1/1 -> If/2
  Compare To Constant4/1 -> If/1
  Unit Delay1/1 -> Exhalation/5(rPatientValveCmdPrev [%])
  [rPatientValveCmd] -> Unit Delay1/1
  Unit Delay2/1 -> Inhalation/5(rBlowerValveCmdPrev [%])
  [rBlowerValveCmd] -> Unit Delay2/1
  Compare To Constant5/1 -> Logical Operator1/1
  Compare To Constant2/1 -> Logical Operator1/2
  Merge/1 -> [rBlowerValveCmd], Data Type Conversion/1
  Merge1/1 -> [rPatientValveCmd], Data Type Conversion1/1
  [pBlowerValveOutlet] -> Inhalation/4(pBlowerValveOutlet [mmH2O])
  [pBlowerValveOutletTarget] -> Inhalation/3(pBlowerValveOutletTarget [mmH2O])
  [tPeriodTask] -> Inhalation/2(tPeriodTask [s])
  Detect Increase1/1 -> Inhalation/1(BExternalInit [-])
  [tPeriodTask] -> Exhalation/2(tPeriodTask [s])
  NRespiratorCycleStatus [-]/1 -> [NRespiratorCycleStatus]
  tPeriodTask [s]/1 -> [tPeriodTask]
  Detect Increase/1 -> Exhalation/1(BExternalInit [-])
  [pBlowerValveOutlet] -> Exhalation/4(pBlowerValveOutlet [mmH2O])
  pBlowerValveOutlet [mmH2O]/1 -> [pBlowerValveOutlet]
  [pBlowerValveOutletTarget] -> Exhalation/3(pBlowerValveOutletTarget [mmH2O])
  pBlowerValveOutletTarget [mmH2O]/1 -> [pBlowerValveOutletTarget]
  [NRespiratorCycleStatus] -> Compare To Constant3/1, Compare To Constant4/1, Compare To Constant1/1, Compare To Constant5/1, Compare To Constant2/1

== system LIB_CycleControl/Cycle Control/Cycle Control Wrapper/Cycle pController/BlowerSpeed_Target/CycleStartComputation ==
  pBlowerValveOutletPlateauLastCycle [mmH2O] : Inport
  tStopInhalationPhase1LastCycle [s] : Inport  Port=2
  tInhalationMaxDurationLastCycle [s] : Inport  Port=3
  "pBlowerValveOutletStaticErrorLastCycle [mmH2O] " : Inport  Port=4
  pBlowerValveOutletErrorMaxLastCycle [mmH2O] : Inport  Port=5
  pDiffBlowerValveOutletTarget [mmH2O] : Inport  Port=6
  nBlowerCmdPrev [rpm] : Inport  Port=7
  Action Port : ActionPort
  Blower Inc from Last Cycle : Subsystem
  Compare To Zero2 : simulink/Logic and Bit Operations/Compare To Zero  relop=>  OutDataTypeStr=boolean
  Constant20 : Constant  Value=nBlowerCmdMax  OutDataTypeStr=single
  Constant21 : Constant  Value=nBlowerCmdMin  OutDataTypeStr=single
  Constant22 : Constant  Value=NBlowerSpeedIncCorrectionGain  OutDataTypeStr=single
  Constant5 : Constant  Value=pErrorPlausibilityThd  OutDataTypeStr=single
  Constant7 : Constant  Value=0  OutDataTypeStr=single
  Data Store Write4 : DataStoreWrite  DataStoreName=nBlowerInc
  Logical Operator1 : Logic  AllPortsSameDT=off  OutDataTypeStr=boolean
  Product1 : Product
  Relational Operator4 : RelationalOperator  Operator=<  OutDataTypeStr=boolean  RndMeth=Simplest
  Saturation Dynamic with flags : Subsystem  mask(Saturation Dynamic){OutMin=[], OutMax=[], OutDataTypeStr=Inherit: Same as second input, OutputDataTypeScalingMode=Same as second input, OutDataType=fixdt(1, 16), OutScaling=2^-10, LockScale=off, RndMeth=Floor, DoSatur=off}
      mask prompts: OutMin "Output minimum:"; OutMax "Output maximum:"; OutDataTypeStr "Output data type:"; OutputDataTypeScalingMode "Output data type mode:"; OutDataType "Output data type (e.g. fixdt(1, 16), fixdt('single')):"; OutScaling "Output scaling (Slope, e.g. 2^-9 or [Slope Bias], e.g. [1.25 3]):"; LockScale "Lock output data type setting against changes by the fixed-point tools"; RndMeth "Integer rounding mode:"; DoSatur "Saturate on integer overflow"
      mask help: Bound the range of the second input by using the first input (upper limit) and the third input (lower limit).
      mask init:
      | blkH = gcbh;
      | blkName = getfullname(blkH);
      | 
      | switch_blks = {'Switch','Switch2'}; 
      | for i = 1:length(switch_blks)
      |   set_param([blkName,'/',switch_blks{i}], ...
      |       'RndMeth', RndMeth, ...
      | 	  'DoSatur', DoSatur);
      | end
      | 
      | propBlk = [blkName, '/Data Type Propagation'];
      | 
      | if strcmp(OutputDataTypeScalingMode, 'Same as second input')
      |     set_param(propBlk, 'PropDataTypeMode', 'Inherit via propagation rule', ...
      |                        'PropScalingMode',  'Inherit via propagation rule');
      | else
      |     scaling = OutScaling;
      |     switch OutputDataTypeScalingMode
      |       case 'double'
      |         dataType = 'fixdt(''double'')';
      |       case 'single'
      |         dataType = 'fixdt(''single'')';
      |       case 'int8'
      |         dataType = 'fixdt(1,8,0)';
      |       case 'uint8'
      |         dataType = 'fixdt(0,8,0)';
      |       case 'int16'
      |         dataType = 'fixdt(1,16,0)';
      |       case 'uint16'
      |         dataType = 'fixdt(0,16,0)';
      |       case 'int32'
      |         dataType = 'fixdt(1,32,0)';
      |       case 'uint32'
      |         dataType = 'fixdt(0,32,0)';
      |       case 'Specify via dialog'
      |         dataType = OutDataType;
      |     end
      |     
      |     set_param(propBlk, 'PropDataTypeMode', 'Specify via dialog', ...
      |                        'PropScalingMode',  'Specify via dialog', ...
      |                        'PropDataType',     dataType, ...
      |                        'PropScaling',      scaling);
      | end
      mask Callback OutDataTypeStr: fixptdialog(gcbh)
      mask TypeOptions OutputDataTypeScalingMode: double | single | int8 | uint8 | int16 | uint16 | int32 | uint32 | Specify via dialog | Same as second input
      mask Callback OutputDataTypeScalingMode: fixptdialog(gcbh)
      mask Callback OutDataType: fixptdialog(gcbh)
      mask TypeOptions RndMeth: Ceiling | Convergent | Floor | Nearest | Round | Simplest | Zero
      mask Display: plot([0.15 0.85],[.5 .5],[.5 .5],[0.05 0.95],0.15+0.7*[0 .25 .75 1],0.05+0.9*[.25 .25 .75 .75]);
  Signal Conversion3 : SignalConversion  OverrideOpt=off
  Sum2 : Sum  Inputs=|++
  Switch6 : Switch  Criteria=u2 ~= 0
      settings: AttributesFormatString=%<Criteria>
  Terminator1 : Terminator
  Terminator2 : Terminator
  nBlowerCmd [rpm] : Outport
  wires:
  Logical Operator1/1 -> Switch6/2
  Relational Operator4/1 -> Logical Operator1/2
  Compare To Zero2/1 -> Logical Operator1/1
  [pBlowerValveOutletErrorMaxLastCycle] -> Relational Operator4/1
  Constant5/1 -> Relational Operator4/2
  tInhalationMaxDurationLastCycle [s]/1 -> Blower Inc from Last Cycle/2(tInhalationMaxDurationLastCycle [s])
  tStopInhalationPhase1LastCycle [s]/1 -> Blower Inc from Last Cycle/1(tStopInhalationPhase1LastCycle [s])
  pBlowerValveOutletErrorMaxLastCycle [mmH2O]/1 -> Blower Inc from Last Cycle/4(pBlowerValveOutletErrorMaxLastCycle [mmH2O]), [pBlowerValveOutletErrorMaxLastCycle]
  pDiffBlowerValveOutletTarget [mmH2O]/1 -> Blower Inc from Last Cycle/5(pDiffBlowerValveOutletTarget [mmH2O])
  Constant22/1 -> Product1/1
  Constant7/1 -> Switch6/3
  Blower Inc from Last Cycle/1(nBlowerInc [rpm]) -> Switch6/1
  pBlowerValveOutletPlateauLastCycle [mmH2O]/1 -> Compare To Zero2/1
  Signal Conversion3/1 -> nBlowerCmd [rpm]/1
  Saturation Dynamic with flags/3(BsatDown [-]) -> Terminator2/1
  Saturation Dynamic with flags/1(BsatUp [-]) -> Terminator1/1
  Saturation Dynamic with flags/2(y) -> Signal Conversion3/1
  Constant21/1 -> Saturation Dynamic with flags/3(lo)
  Constant20/1 -> Saturation Dynamic with flags/1(up)
  Product1/1 -> Sum2/2, Data Store Write4/1  "nBlowerInc"
  Sum2/1 -> Saturation Dynamic with flags/2(u)
  nBlowerCmdPrev [rpm]/1 -> Sum2/1
  "pBlowerValveOutletStaticErrorLastCycle [mmH2O] "/1 -> Blower Inc from Last Cycle/3("pBlowerValveOutletStaticErrorLastCycle [mmH2O] ")
  Switch6/1 -> Product1/2

== system LIB_CycleControl/Cycle Control/Cycle Control Wrapper/Cycle pController/BlowerSpeed_Target/START ==
  tCycle [s] : Inport
  Action Port : ActionPort
  Constant13 : Constant  Value=nBlowerCmdInit  OutDataTypeStr=single
  Constant4 : Constant  Value=tDelayBeforeRespiratorCycleStart  OutDataTypeStr=single
  Constant9 : Constant  Value=0  OutDataTypeStr=single
  Gain : Gain  Gain=0.5
  Relational Operator : RelationalOperator  Operator=>  OutDataTypeStr=boolean  RndMeth=Simplest
  Switch3 : Switch  Criteria=u2 ~= 0
      settings: AttributesFormatString=%<Criteria>
  nBlowerCmd [rpm] : Outport
  wires:
  Constant4/1 -> Gain/1
  Constant13/1 -> Switch3/1
  Gain/1 -> Relational Operator/2
  Switch3/1 -> nBlowerCmd [rpm]/1
  Constant9/1 -> Switch3/3
  Relational Operator/1 -> Switch3/2
  tCycle [s]/1 -> Relational Operator/1

== system LIB_CycleControl/Cycle Control/Cycle Control Wrapper/Cycle pController/BlowerSpeed_Target/STOP ==
  Action Port : ActionPort
  Constant9 : Constant  Value=0  OutDataTypeStr=single
  nBlowerCmd [rpm] : Outport
  wires:
  Constant9/1 -> nBlowerCmd [rpm]/1

== system LIB_CycleControl/Cycle Control/Cycle Control Wrapper/Cycle pController/Cycle Manager/Timing Setup ==
  NCyclePerMin [-/min] : Inport
  rInhalationPerCycle [-] : Inport  Port=2
  function : TriggerPort  TriggerType=function-call  VariantControl=Variant
  Data Store Write1 : DataStoreWrite  DataStoreName=tInhalationMaxDuration
  Data Store Write2 : DataStoreWrite  DataStoreName=tInhalationMaxDurationLastCycle
  Data Store Write4 : DataStoreWrite  DataStoreName=tCycleMaxDuration
  Timing Setup : Subsystem
  tCycleMaxDuration [s] : Outport
  tInhalationMaxDuration [s] : Outport  Port=2
  tInhalationMaxDurationLastCycle [s] : Outport  Port=3
  wires:
  Timing Setup/3(tInhalationMaxDurationLastCycle [s]) -> tInhalationMaxDurationLastCycle [s]/1, Data Store Write2/1  "tInhalationMaxDurationLastCycle"
  Timing Setup/2(tInhalationMaxDuration [s]) -> tInhalationMaxDuration [s]/1, Data Store Write1/1  "tInhalationMaxDuration"
  Timing Setup/1(tCycleMaxDuration [s]) -> tCycleMaxDuration [s]/1, Data Store Write4/1  "tCycleMaxDuration"
  rInhalationPerCycle [-]/1 -> Timing Setup/2(rInhalationPerCycle)
  NCyclePerMin [-/min]/1 -> Timing Setup/1(NCyclePerMin [-/min])

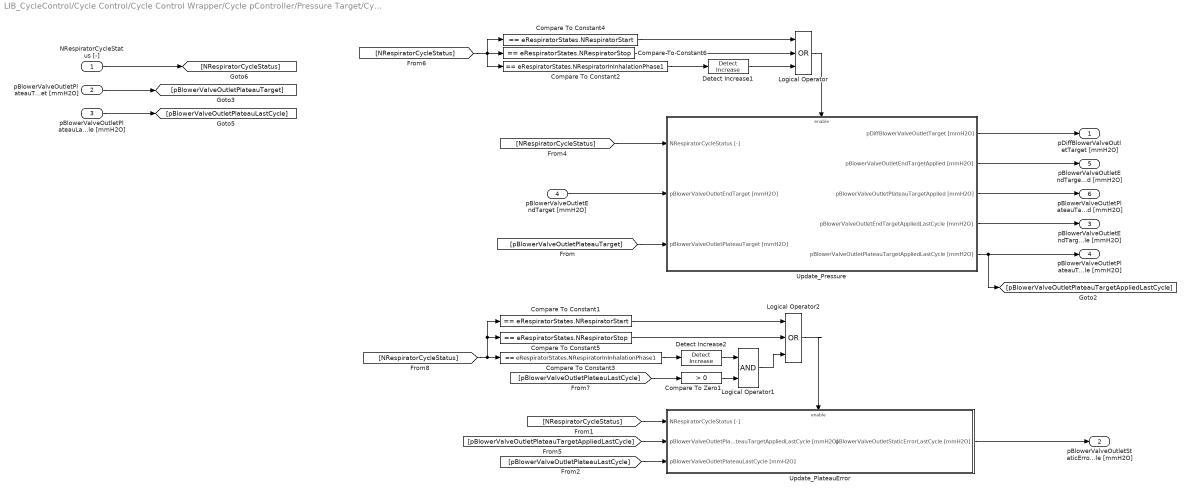
== system LIB_CycleControl/Cycle Control/Cycle Control Wrapper/Cycle pController/Pressure Target/CycleStartComputation ==
  NRespiratorCycleStatus [-] : Inport
  pBlowerValveOutletPlateauTarget [mmH2O] : Inport  Port=2
  pBlowerValveOutletPlateauLastCycle [mmH2O] : Inport  Port=3
  pBlowerValveOutletEndTarget [mmH2O] : Inport  Port=4
  Compare To Constant1 : simulink/Logic and Bit Operations/Compare To Constant  relop===  const=eRespiratorStates.NRespiratorStart  OutDataTypeStr=boolean
  Compare To Constant2 : simulink/Logic and Bit Operations/Compare To Constant  relop===  const=eRespiratorStates.NRespiratorInInhalationPhase1  OutDataTypeStr=boolean
  Compare To Constant3 : simulink/Logic and Bit Operations/Compare To Constant  relop===  const=eRespiratorStates.NRespiratorInInhalationPhase1  OutDataTypeStr=boolean
  Compare To Constant4 : simulink/Logic and Bit Operations/Compare To Constant  relop===  const=eRespiratorStates.NRespiratorStart  OutDataTypeStr=boolean
  Compare To Constant5 : simulink/Logic and Bit Operations/Compare To Constant  relop===  const=eRespiratorStates.NRespiratorStop  OutDataTypeStr=boolean
  Compare To Constant6 : simulink/Logic and Bit Operations/Compare To Constant  relop===  const=eRespiratorStates.NRespiratorStop  OutDataTypeStr=boolean
  Compare To Zero1 : simulink/Logic and Bit Operations/Compare To Zero  relop=>  OutDataTypeStr=boolean
  Detect Increase1 : simulink/Logic and Bit Operations/Detect Increase  vinit=0.0  OutDataTypeStr=boolean
  Detect Increase2 : simulink/Logic and Bit Operations/Detect Increase  vinit=0.0  OutDataTypeStr=boolean
  Logical Operator : Logic  Operator=OR  Inputs=3  AllPortsSameDT=off  OutDataTypeStr=boolean
  Logical Operator1 : Logic  AllPortsSameDT=off  OutDataTypeStr=boolean
  Logical Operator2 : Logic  Operator=OR  Inputs=3  AllPortsSameDT=off  OutDataTypeStr=boolean
  Update_PlateauError : Subsystem
  Update_Pressure : Subsystem
  pDiffBlowerValveOutletTarget [mmH2O] : Outport
  pBlowerValveOutletStaticErrorLastCycle [mmH2O] : Outport  Port=2
  pBlowerValveOutletEndTargetAppliedLastCycle [mmH2O] : Outport  Port=3
  pBlowerValveOutletPlateauTargetAppliedLastCycle [mmH2O] : Outport  Port=4
  pBlowerValveOutletEndTargetApplied [mmH2O] : Outport  Port=5
  pBlowerValveOutletPlateauTargetApplied [mmH2O] : Outport  Port=6
  wires:
  Update_Pressure/4(pBlowerValveOutletEndTargetAppliedLastCycle [mmH2O]) -> pBlowerValveOutletEndTargetAppliedLastCycle [mmH2O]/1
  Update_Pressure/1(pDiffBlowerValveOutletTarget [mmH2O]) -> pDiffBlowerValveOutletTarget [mmH2O]/1
  Update_PlateauError/1(pBlowerValveOutletStaticErrorLastCycle [mmH2O]) -> pBlowerValveOutletStaticErrorLastCycle [mmH2O]/1
  [pBlowerValveOutletPlateauTargetAppliedLastCycle] -> Update_PlateauError/2(pBlowerValveOutletPlateauTargetAppliedLastCycle [mmH2O])
  Update_Pressure/5(pBlowerValveOutletPlateauTargetAppliedLastCycle [mmH2O]) -> [pBlowerValveOutletPlateauTargetAppliedLastCycle], pBlowerValveOutletPlateauTargetAppliedLastCycle [mmH2O]/1
  Detect Increase2/1 -> Logical Operator1/1
  [NRespiratorCycleStatus] -> Compare To Constant3/1, Compare To Constant5/1, Compare To Constant1/1
  Compare To Constant3/1 -> Detect Increase2/1
  Update_Pressure/3(pBlowerValveOutletPlateauTargetApplied [mmH2O]) -> pBlowerValveOutletPlateauTargetApplied [mmH2O]/1
  Update_Pressure/2(pBlowerValveOutletEndTargetApplied [mmH2O]) -> pBlowerValveOutletEndTargetApplied [mmH2O]/1
  Logical Operator/1 -> Update_Pressure/Enable
  Compare To Constant4/1 -> Logical Operator/1
  [pBlowerValveOutletPlateauTarget] -> Update_Pressure/3(pBlowerValveOutletPlateauTarget [mmH2O])
  pBlowerValveOutletEndTarget [mmH2O]/1 -> Update_Pressure/2(pBlowerValveOutletEndTarget [mmH2O])
  [NRespiratorCycleStatus] -> Compare To Constant2/1, Compare To Constant6/1, Compare To Constant4/1
  Compare To Constant2/1 -> Detect Increase1/1
  NRespiratorCycleStatus [-]/1 -> [NRespiratorCycleStatus]
  Compare To Zero1/1 -> Logical Operator1/2
  [pBlowerValveOutletPlateauLastCycle] -> Update_PlateauError/3(pBlowerValveOutletPlateauLastCycle [mmH2O])
  [pBlowerValveOutletPlateauLastCycle] -> Compare To Zero1/1
  pBlowerValveOutletPlateauLastCycle [mmH2O]/1 -> [pBlowerValveOutletPlateauLastCycle]
  pBlowerValveOutletPlateauTarget [mmH2O]/1 -> [pBlowerValveOutletPlateauTarget]
  Compare To Constant1/1 -> Logical Operator2/1
  Logical Operator1/1 -> Logical Operator2/3
  Logical Operator2/1 -> Update_PlateauError/Enable
  Compare To Constant5/1 -> Logical Operator2/2
  [NRespiratorCycleStatus] -> Update_PlateauError/1(NRespiratorCycleStatus [-])
  Compare To Constant6/1 -> Logical Operator/2
  [NRespiratorCycleStatus] -> Update_Pressure/1(NRespiratorCycleStatus [-])
  Detect Increase1/1 -> Logical Operator/3

== system LIB_CycleControl/Cycle Control/Cycle Control Wrapper/Cycle pController/Pressure Target/InCycleComputation ==
  NRespiratorCycleStatus [-] : Inport
  pBlowerValveOutletEndTargetApplied [mmH2O] : Inport  Port=2
  pBlowerValveOutletPlateauTargetApplied [mmH2O] : Inport  Port=3
  Compare To Constant1 : simulink/Logic and Bit Operations/Compare To Constant  relop===  const=eRespiratorStates.NRespiratorStart  OutDataTypeStr=boolean
  Compare To Constant2 : simulink/Logic and Bit Operations/Compare To Constant  relop===  const=eRespiratorStates.NRespiratorInInhalationPhase2  OutDataTypeStr=boolean
  Compare To Constant3 : simulink/Logic and Bit Operations/Compare To Constant  relop===  const=eRespiratorStates.NRespiratorStop  OutDataTypeStr=boolean
  Compare To Constant4 : simulink/Logic and Bit Operations/Compare To Constant  relop===  const=eRespiratorStates.NRespiratorInExhalation  OutDataTypeStr=boolean
  Compare To Constant5 : simulink/Logic and Bit Operations/Compare To Constant  relop===  const=eRespiratorStates.NRespiratorInInhalationPhase1  OutDataTypeStr=boolean
  Detect Increase1 : simulink/Logic and Bit Operations/Detect Increase  vinit=0.0  OutDataTypeStr=boolean
  Detect Increase2 : simulink/Logic and Bit Operations/Detect Increase  vinit=0.0  OutDataTypeStr=boolean
  Detect Increase3 : simulink/Logic and Bit Operations/Detect Increase  vinit=0.0  OutDataTypeStr=boolean
  Logical Operator : Logic  Operator=OR  Inputs=5  AllPortsSameDT=off  OutDataTypeStr=boolean
  UpdatePressureTarget : Subsystem
  pBlowerValveOutletTarget [mmH2O] : Outport
  wires:
  Logical Operator/1 -> UpdatePressureTarget/Enable
  Detect Increase1/1 -> Logical Operator/2
  Detect Increase3/1 -> Logical Operator/4
  Compare To Constant4/1 -> Detect Increase3/1
  Detect Increase2/1 -> Logical Operator/3
  NRespiratorCycleStatus [-]/1 -> UpdatePressureTarget/1(NRespiratorCycleStatus [-]), Compare To Constant3/1, Compare To Constant1/1, Compare To Constant5/1, Compare To Constant2/1, Compare To Constant4/1
  Compare To Constant2/1 -> Detect Increase2/1
  Compare To Constant1/1 -> Logical Operator/1
  Compare To Constant5/1 -> Detect Increase1/1
  UpdatePressureTarget/1(pBlowerValveOutletTarget [mmH2O]) -> pBlowerValveOutletTarget [mmH2O]/1
  pBlowerValveOutletPlateauTargetApplied [mmH2O]/1 -> UpdatePressureTarget/3(pBlowerValveOutletPlateauTargetApplied [mmH2O])
  pBlowerValveOutletEndTargetApplied [mmH2O]/1 -> UpdatePressureTarget/2(pBlowerValveOutletEndTargetApplied [mmH2O])
  Compare To Constant3/1 -> Logical Operator/5

== system LIB_CycleControl/Cycle Control/Cycle Control Wrapper/Cycle pController/Pressure processing/PPeak Computation ==
  BInitCyclePressure [-] : Inport
  NRespiratorCycleStatus [-] : Inport  Port=2
  pBlowerValveOutlet [mmH2O] : Inport  Port=3
  Compare To Constant1 : simulink/Logic and Bit Operations/Compare To Constant  relop===  const=eRespiratorStates.NRespiratorInInhalationPhase1  OutDataTypeStr=boolean
  Compare To Constant6 : simulink/Logic and Bit Operations/Compare To Constant  relop===  const=eRespiratorStates.NRespiratorInInhalationPhase2  OutDataTypeStr=boolean
  Data Store Write3 : DataStoreWrite  DataStoreName=pBlowerValveOutletPeakCurrent
  Logical Operator : Logic  Operator=OR  Inputs=3  AllPortsSameDT=off  OutDataTypeStr=boolean
  Peak Monitoring : Subsystem
  Unit Delay : UnitDelay  SampleTime=-1
      settings: AttributesFormatString=%<InitialCondition>
  pBlowerValveOutletPeakCurrent [mmH2O] : Outport  OutDataTypeStr=single
  wires:
  BInitCyclePressure [-]/1 -> [BInitCyclePressure]
  Peak Monitoring/1(pBlowerValveOutletPeakCurrent [mmH2O]) -> Unit Delay/1, pBlowerValveOutletPeakCurrent [mmH2O]/1, Data Store Write3/1  "pBlowerValveOutletPeakCurrent"
  pBlowerValveOutlet [mmH2O]/1 -> [pBlowerValveOutlet]
  NRespiratorCycleStatus [-]/1 -> [NRespiratorCycleStatus]
  [pBlowerValveOutlet] -> Peak Monitoring/2(pBlowerValveOutlet [mmH2O])
  Logical Operator/1 -> Peak Monitoring/Enable
  [NRespiratorCycleStatus] -> Compare To Constant1/1, Compare To Constant6/1
  Compare To Constant6/1 -> Logical Operator/3
  [BInitCyclePressure] -> Logical Operator/1
  Compare To Constant1/1 -> Logical Operator/2
  Unit Delay/1 -> Peak Monitoring/3(pBlowerValveOutletPeakCurrentPrev [mmH2O])
  [BInitCyclePressure] -> Peak Monitoring/1(BInitCyclePressure [-])
